simulink model "simL0_multiPath"  (R2024a)
settings: Solver=ode4  StartTime=0.0  StopTime=1500  FixedStep=0.01  MaxStep=0.01  MinStep=10^-3  RelTol=0.01
values from neighbouring files (symbols this model uses):
  MegAWESkite = yaml.ReadYaml('MegAWESkite.yaml',false,true)    [runMain.m]
undefined symbols (not defined in the file or in its folder): actuatorLimit, controllerGains_retraction, controllerGains_traction, DiscIntNeverNeededParam, ENVMT, pathparam, simInit, tetherParams, winchParameter
libraries: simulink x9, slpidlib x9, sharedtransform x3, aerolibutil x3, dspswit3 x2, dspinverses x2, shared6dof x1, simulink_extras x1, dspsigops x1, dspstat3 x1, vrlib x1
(part 5 of 5)

== matlab function simL0_multiPath/Output/Convergence_check/MATLAB Function2 ==
  settings: updateMethod=DISCRETE  sampleTime=simInit.Ts_power_conv_check
  data: flag input; m_old input; p_sum input; cnt input; u input; flag output; flightMode input; e_old input; cnt_max_mat input; cycles_cnt input; m_new output; p_sum output; cnt output; e_new output; cnt_max_mat output; cycles_cnt output
% Copyright 2021 Delft University of Technology
%
% Licensed under the Apache License, Version 2.0 (the "License");
% you may not use this file except in compliance with the License.
% You may obtain a copy of the License at
%
%      http://www.apache.org/licenses/LICENSE-2.0
%
% Unless required by applicable law or agreed to in writing, software
% distributed under the License is distributed on an "AS IS" BASIS,
% WITHOUT WARRANTIES OR CONDITIONS OF ANY KIND, either express or implied.
% See the License for the specific language governing permissions and
% limitations under the License.

function [flag, m_new, p_sum, cnt, e_new, cnt_max_mat,cycles_cnt] = fcn(flag, m_old, p_sum, cnt, u, flightMode, e_old,cnt_max_mat,cycles_cnt)

p_sum = p_sum + u;
cnt = cnt + 1;

if (flightMode == 1) && flag % traction
    cnt_max_mat = cnt; 
    m_new = p_sum/cnt;
    cnt  = 0;
    cycles_cnt = cycles_cnt + 1;
    p_sum = 0;
    flag = 0;
    e_new = abs( m_new - m_old );
elseif (flightMode == 2 || flightMode == 3) % retraction & transition
    flag = 1;
    m_new = m_old;
    e_new = e_old;
else
    flag = 0;
    m_new = m_old;
    e_new = e_old;
end

end
